simulink model "SWC_FDC_type"  (R2021b)
settings: Solver=FixedStepDiscrete  StartTime=0.0  StopTime=10.0  FixedStep=0.001  RelTol=1e-3
values from neighbouring files (symbols this model uses):
  C_TASK_5MS_S = (	C_TICK_TIME_S      	)    [vcu_local_hdr.m]
  DID_VCUKey = uint16(0x0202)    [vcu_local_hdr.m]
  DID_XWD = uint16(513)    [vcu_local_hdr.m]
  DIDLen_DKCKey = uint16(8)    [vcu_local_hdr.m]
  DIDLen_FoxPiBattSta = uint16(4)    [vcu_local_hdr.m]
  DIDLen_FoxPiBrakeSta = uint16(13)    [vcu_local_hdr.m]
  DIDLen_FoxPiButtonSta = uint16(2)    [vcu_local_hdr.m]
  DIDLen_FoxPiCtrlEnSw = uint16(1)    [vcu_local_hdr.m]
  DIDLen_FoxPiDrivingCtrl = uint16(21)    [vcu_local_hdr.m]
  DIDLen_FoxPiEPSSta = uint16(11)    [vcu_local_hdr.m]
  DIDLen_FoxPiLampCtrl = uint16(6)    [vcu_local_hdr.m]
  DIDLen_FoxPiLampSta = uint16(2)    [vcu_local_hdr.m]
  DIDLen_FoxPiMotionSta = uint16(13)    [vcu_local_hdr.m]
  DIDLen_FoxPiMotorSta = uint16(11)    [vcu_local_hdr.m]
  DIDLen_FoxPiPedalPos = uint16(3)    [vcu_local_hdr.m]
  DIDLen_FoxPiPTGUSSSw = uint16(1)    [vcu_local_hdr.m]
  DIDLen_FoxPiShifterAllow = uint16(3)    [vcu_local_hdr.m]
  DIDLen_FoxPiSwSta = uint16(2)    [vcu_local_hdr.m]
  DIDLen_FoxPiTPMSSta = uint16(13)    [vcu_local_hdr.m]
  DIDLen_FoxPiUSSDist = uint16(20)    [vcu_local_hdr.m]
  DIDLen_FoxPiUSSFaultSta = uint16(2)    [vcu_local_hdr.m]
  DIDLen_FoxPiWheelSpd = uint16(16)    [vcu_local_hdr.m]
  DIDNum_DKCKey = uint16(0x0202)    [vcu_local_hdr.m]
  DIDNum_FoxPiBattSta = uint16(0x100D)    [vcu_local_hdr.m]
  DIDNum_FoxPiBrakeSta = uint16(0x1003)    [vcu_local_hdr.m]
  DIDNum_FoxPiButtonSta = uint16(0x1006)    [vcu_local_hdr.m]
  DIDNum_FoxPiCtrlEnSw = uint16(0x1012)    [vcu_local_hdr.m]
  DIDNum_FoxPiDrivingCtrl = uint16(0x1001)    [vcu_local_hdr.m]
  DIDNum_FoxPiEPSSta = uint16(0x1005)    [vcu_local_hdr.m]
  DIDNum_FoxPiLampCtrl = uint16(0x100C)    [vcu_local_hdr.m]
  DIDNum_FoxPiLampSta = uint16(0x100B)    [vcu_local_hdr.m]
  DIDNum_FoxPiMotionSta = uint16(0x1002)    [vcu_local_hdr.m]
  DIDNum_FoxPiMotorSta = uint16(0x1010)    [vcu_local_hdr.m]
  DIDNum_FoxPiPedalPos = uint16(0x100F)    [vcu_local_hdr.m]
  DIDNum_FoxPiPTGUSSSw = uint16(0x1009)    [vcu_local_hdr.m]
  DIDNum_FoxPiShifterAllow = uint16(0x1011)    [vcu_local_hdr.m]
  DIDNum_FoxPiSwSta = uint16(0x100A)    [vcu_local_hdr.m]
  DIDNum_FoxPiTPMSSta = uint16(0x100E)    [vcu_local_hdr.m]
  DIDNum_FoxPiUSSDist = uint16(0x1007)    [vcu_local_hdr.m]
  DIDNum_FoxPiUSSFaultSta = uint16(0x1008)    [vcu_local_hdr.m]
  DIDNum_FoxPiWheelSpd = uint16(0x1004)    [vcu_local_hdr.m]
  DIDVCUKeyLength = uint16(8)    [vcu_local_hdr.m]
  DTC_10020B = Simulink.Parameter    [DTC_Constant_Definition.m]
  DTC_10020C = Simulink.Parameter    [DTC_Constant_Definition.m]
  DTC_10020D = Simulink.Parameter    [DTC_Constant_Definition.m]
  DTC_10020E = Simulink.Parameter    [DTC_Constant_Definition.m]
  DTC_100210 = Simulink.Parameter    [DTC_Constant_Definition.m]
  DTC_100211 = Simulink.Parameter    [DTC_Constant_Definition.m]
  DTC_100212 = Simulink.Parameter    [DTC_Constant_Definition.m]
  DTC_100213 = Simulink.Parameter    [DTC_Constant_Definition.m]
  DTC_100214 = Simulink.Parameter    [DTC_Constant_Definition.m]
  DTC_100215 = Simulink.Parameter    [DTC_Constant_Definition.m]
  DTC_100216 = Simulink.Parameter    [DTC_Constant_Definition.m]
  DTC_100217 = Simulink.Parameter    [DTC_Constant_Definition.m]
  DTC_100218 = Simulink.Parameter    [DTC_Constant_Definition.m]
  DTC_100219 = Simulink.Parameter    [DTC_Constant_Definition.m]
  DTC_10021A = Simulink.Parameter    [DTC_Constant_Definition.m]
  DTC_10021B = Simulink.Parameter    [DTC_Constant_Definition.m]
  DTC_10021C = Simulink.Parameter    [DTC_Constant_Definition.m]
  DTC_10021D = Simulink.Parameter    [DTC_Constant_Definition.m]
  DTC_10021E = Simulink.Parameter    [DTC_Constant_Definition.m]
  DTC_100220 = Simulink.Parameter    [DTC_Constant_Definition.m]
  DTC_100221 = Simulink.Parameter    [DTC_Constant_Definition.m]
  DTC_100223 = Simulink.Parameter    [DTC_Constant_Definition.m]
  DTC_100224 = Simulink.Parameter    [DTC_Constant_Definition.m]
  DTC_100225 = Simulink.Parameter    [DTC_Constant_Definition.m]
  DTC_100226 = Simulink.Parameter    [DTC_Constant_Definition.m]
  DTC_100227 = Simulink.Parameter    [DTC_Constant_Definition.m]
  DTC_100242 = Simulink.Parameter    [DTC_Constant_Definition.m]
  DTC_100243 = Simulink.Parameter    [DTC_Constant_Definition.m]
  DTC_100244 = Simulink.Parameter    [DTC_Constant_Definition.m]
  DTC_100247 = Simulink.Parameter    [DTC_Constant_Definition.m]
  DTC_100248 = Simulink.Parameter    [DTC_Constant_Definition.m]
  DTC_100249 = Simulink.Parameter    [DTC_Constant_Definition.m]
  DTC_100250 = Simulink.Parameter    [DTC_Constant_Definition.m]
  DTC_100251 = Simulink.Parameter    [DTC_Constant_Definition.m]
  DTC_100252 = Simulink.Parameter    [DTC_Constant_Definition.m]
  DTC_100A10 = Simulink.Parameter    [DTC_Constant_Definition.m]
  DTC_100A12 = Simulink.Parameter    [DTC_Constant_Definition.m]
  DTC_100A16 = Simulink.Parameter    [DTC_Constant_Definition.m]
  DTC_100A17 = Simulink.Parameter    [DTC_Constant_Definition.m]
  DTC_100A18 = Simulink.Parameter    [DTC_Constant_Definition.m]
  DTC_100A19 = Simulink.Parameter    [DTC_Constant_Definition.m]
  DTC_500B01 = Simulink.Parameter    [DTC_Constant_Definition.m]
  DTC_500B02 = Simulink.Parameter    [DTC_Constant_Definition.m]
  DTC_500B03 = Simulink.Parameter    [DTC_Constant_Definition.m]
  DTC_500B04 = Simulink.Parameter    [DTC_Constant_Definition.m]
  DTC_500B05 = Simulink.Parameter    [DTC_Constant_Definition.m]
  DTC_500B06 = Simulink.Parameter    [DTC_Constant_Definition.m]
  DTC_500B07 = Simulink.Parameter    [DTC_Constant_Definition.m]
  DTC_500B08 = Simulink.Parameter    [DTC_Constant_Definition.m]
  DTC_500B09 = Simulink.Parameter    [DTC_Constant_Definition.m]
  DTC_500B0A = Simulink.Parameter    [DTC_Constant_Definition.m]
  DTC_500B0B = Simulink.Parameter    [DTC_Constant_Definition.m]
  DTC_500B0C = Simulink.Parameter    [DTC_Constant_Definition.m]
  DTC_500B0D = Simulink.Parameter    [DTC_Constant_Definition.m]
  DTC_500B0E = Simulink.Parameter    [DTC_Constant_Definition.m]
  DTC_500B0F = Simulink.Parameter    [DTC_Constant_Definition.m]
  DTC_500B10 = Simulink.Parameter    [DTC_Constant_Definition.m]
  DTC_90021F = Simulink.Parameter    [DTC_Constant_Definition.m]
  DTC_90022F = Simulink.Parameter    [DTC_Constant_Definition.m]
  DTC_900253 = Simulink.Parameter    [DTC_Constant_Definition.m]
  DTC_900254 = Simulink.Parameter    [DTC_Constant_Definition.m]
  DTC_900301 = Simulink.Parameter    [DTC_Constant_Definition.m]
  DTC_900302 = Simulink.Parameter    [DTC_Constant_Definition.m]
  DTC_900303 = Simulink.Parameter    [DTC_Constant_Definition.m]
  DTC_900304 = Simulink.Parameter    [DTC_Constant_Definition.m]
  DTC_900305 = Simulink.Parameter    [DTC_Constant_Definition.m]
  DTC_900909 = Simulink.Parameter    [DTC_Constant_Definition.m]
  DTC_90090A = Simulink.Parameter    [DTC_Constant_Definition.m]
  DTC_90090B = Simulink.Parameter    [DTC_Constant_Definition.m]
  DTC_90090C = Simulink.Parameter    [DTC_Constant_Definition.m]
  DTC_90090D = Simulink.Parameter    [DTC_Constant_Definition.m]
  DTC_90090E = Simulink.Parameter    [DTC_Constant_Definition.m]
  DTC_90090F = Simulink.Parameter    [DTC_Constant_Definition.m]
  DTC_900910 = Simulink.Parameter    [DTC_Constant_Definition.m]
  DTC_900911 = Simulink.Parameter    [DTC_Constant_Definition.m]
  DTC_900912 = Simulink.Parameter    [DTC_Constant_Definition.m]
  DTC_900913 = Simulink.Parameter    [DTC_Constant_Definition.m]
  DTC_900914 = Simulink.Parameter    [DTC_Constant_Definition.m]
  ... (+54 more)
undefined symbols (not defined in the file or in its folder): f32_ApsOutVehSpdSig, KHAL_CANBusOffDebounce_cnt, KHAL_CANBusOffDebounce_s, KHAL_DKCDecryptEnable_flg_ovrdflg, KHAL_DKCDecryptEnable_flg_ovrdval, KHAL_RandomNumberY1_enum, KHAL_RandomNumberY2_enum, KHAL_RandomNumberY_ovrdflg, KHAL_TPMSRESBUTT_flg_ovrdflg, KHAL_TPMSRESBUTT_flg_ovrdval, KINP_ReadVinCode_flg, P_boolean, R_DIDWriteCDD_CSOP_DIDSet_DKCKey, R_DIDWriteCDD_CSOP_DIDSet_FoxPiBattSta, R_DIDWriteCDD_CSOP_DIDSet_FoxPiBrakeSta, R_DIDWriteCDD_CSOP_DIDSet_FoxPiButtonSta, R_DIDWriteCDD_CSOP_DIDSet_FoxPiCtrlEnSw, R_DIDWriteCDD_CSOP_DIDSet_FoxPiDrivingCtrl, R_DIDWriteCDD_CSOP_DIDSet_FoxPiEPSSta, R_DIDWriteCDD_CSOP_DIDSet_FoxPiLampCtrl, R_DIDWriteCDD_CSOP_DIDSet_FoxPiLampSta, R_DIDWriteCDD_CSOP_DIDSet_FoxPiMotionSta, R_DIDWriteCDD_CSOP_DIDSet_FoxPiMotorSta, R_DIDWriteCDD_CSOP_DIDSet_FoxPiPedalPos, R_DIDWriteCDD_CSOP_DIDSet_FoxPiPTGUSSSw, R_DIDWriteCDD_CSOP_DIDSet_FoxPiShifterAllow, R_DIDWriteCDD_CSOP_DIDSet_FoxPiSwSta, R_DIDWriteCDD_CSOP_DIDSet_FoxPiTPMSSta, R_DIDWriteCDD_CSOP_DIDSet_FoxPiUSSDist, R_DIDWriteCDD_CSOP_DIDSet_FoxPiUSSFaultSta, R_DIDWriteCDD_CSOP_DIDSet_FoxPiWheelSpd, R_E2E_CAN3_VCU1_CSOP_Write_CAN3_VCU1, R_E2E_CAN3_VCU1_toNIDEC_CSOP_Write_CAN3_VCU1_toNIDEC, R_E2E_CAN4_VCU1_CSOP_Write_CAN4_VCU1, R_FDCCDD_Inner_CSOP_FDC_AppCallSleep, R_HALIN_IMU_CSOP_IMUSetSta, R_HALINCDD_CSOP_PAS_Handler, R_HALINCDD_CSOP_ResetPedalZeroPosDone, R_HALINCDD_CSOP_TPMSSensorIDRegSetResults, R_HALINCDD_CSOP_UDS_Main, R_HALOUT_APS_CSOP_ApsOutput, R_HALOUTCDD_CSOP_AppNmStateReq, R_HALOUTCDD_CSOP_IVIReset, R_HALOUTCDD_CSOP_SetAcoreRebootCmdACK, R_HALOUTCDD_CSOP_SetSysPwrStat ... (+80)
libraries: FVT_lib x447, simulink x289, hcu_lib x19, hdlsllib x9, app x1, halin x1, halout x1, matrix_library x1, inp x1, outp x1
(part 4 of 15)

== system SWC_FDC_type/run_SWC_FDC_Tx_1000ms_sys ==
  IRV_ms1000_CAN3_SG_GW_IVI6_toNIDEC_read : Inport
  function : TriggerPort  TriggerType=function-call  VariantControl=(inherit)  SampleTimeType=periodic  SampleTime=-1
  P_CAN3_GW_IVI6_toNIDEC_CAN3_SG_GW_IVI6_toNIDEC_write : Outport
  wires:
  IRV_ms1000_CAN3_SG_GW_IVI6_toNIDEC_read/1 -> P_CAN3_GW_IVI6_toNIDEC_CAN3_SG_GW_IVI6_toNIDEC_write/1

== system SWC_FDC_type/run_SWC_FDC_Tx_100ms_sys ==
  IRV_ms100_CAN1_SG_FD1_THCM1_read : Inport
  IRV_ms100_CAN3_SG_FD3_THCM1_read : Inport  Port=2
  function : TriggerPort  TriggerType=function-call  VariantControl=(inherit)  SampleTimeType=periodic  SampleTime=-1
  P_CAN1_FD1_THCM1_CAN1_SG_FD1_THCM1_write : Outport
  P_CAN3_FD3_THCM1_CAN3_SG_FD3_THCM1_write : Outport  Port=2
  wires:
  IRV_ms100_CAN1_SG_FD1_THCM1_read/1 -> P_CAN1_FD1_THCM1_CAN1_SG_FD1_THCM1_write/1
  IRV_ms100_CAN3_SG_FD3_THCM1_read/1 -> P_CAN3_FD3_THCM1_CAN3_SG_FD3_THCM1_write/1

== system SWC_FDC_type/run_SWC_FDC_Tx_10ms_sys ==
  IRV_ms10_CAN1_SG_FD1_APS3_read : Inport
  IRV_ms10_CAN1_SG_FD1_VCU2_read : Inport  Port=2
  IRV_ms10_CAN1_SG_FD1_VCU3_read : Inport  Port=3
  IRV_ms10_CAN1_SG_VMC_FCM1_read : Inport  Port=4
  IRV_ms10_CAN3_SG_FD3_VCU0_read : Inport  Port=5
  IRV_ms10_CAN3_SG_FD3_VCU2_read : Inport  Port=6
  IRV_ms10_CAN3_SG_FD3_VCU2_toNIDEC_read : Inport  Port=7
  IRV_ms10_CAN3_SG_FD3_VCU5_read : Inport  Port=8
  IRV_ms10_CAN3_SG_GW_ESC1_toNIDEC_read : Inport  Port=9
  IRV_ms10_CAN5_SG_FD5_Debug3_read : Inport  Port=10
  IRV_ms10_CAN6_SG_FD6_APS3_read : Inport  Port=11
  IRV_ms10_CAN6_SG_FD6_VCU2_read : Inport  Port=12
  IRV_f32_ApsOutVehSpdSig_read : Inport  Port=13
  IRV_u8_ApsOutGearPosnSig_read : Inport  Port=14
  IRV_u8_ApsOutSendChrgPlugSta_read : Inport  Port=15
  IRV_u8_ApsOutSetFrSensorOnCmd_read : Inport  Port=16
  IRV_u8_ApsOutSetFrSensorSwTOCmd_read : Inport  Port=17
  IRV_u8_ApsOutSetVehSpdTOCmd_read : Inport  Port=18
  function : TriggerPort  TriggerType=function-call  VariantControl=(inherit)  SampleTimeType=periodic  SampleTime=-1
  R_HALINCDD_CSOP_TPMS_GetRawData : FunctionCaller  FunctionPrototype=[u8_TPMSDataInSta,u8Array9_TPMSData] = R_HALINCDD_CSOP_TPMS_GetRawData()  OutputArgumentSpecifications=P_boolean, uint8([1;1;1;1;1;1;1;1;1])
  R_HALIN_APS_CSOP_ApsGetDist : FunctionCaller  FunctionPrototype=[u8Array8_PasInDist,u16Array4_ApsInDist] = R_HALIN_APS_CSOP_ApsGetDist()  OutputArgumentSpecifications=uint8([1;1;1;1;1;1;1;1]), uint16([1;1;1;1])
  R_HALIN_APS_CSOP_ApsGetDistLevel : FunctionCaller  FunctionPrototype=u8Array8_ApsInLevel = R_HALIN_APS_CSOP_ApsGetDistLevel()  OutputArgumentSpecifications=uint8([1;1;1;1;1;1;1;1])
  R_HALIN_APS_CSOP_ApsGetOtherStatus : FunctionCaller  FunctionPrototype=[u8_ApsInPASChime,u8_ApsInSensorLayout,u8_ApsInSysFailSta,u8_ApsInSysMode] = R_HALIN_APS_CSOP_ApsGetOtherStatus()  OutputArgumentSpecifications=uint8(1), uint8(1), uint8(1), uint8(1)
  R_HALIN_APS_CSOP_ApsGetUssSta : FunctionCaller  FunctionPrototype=u8Array12_ApsInUssSta = R_HALIN_APS_CSOP_ApsGetUssSta()  OutputArgumentSpecifications=uint8([1;1;1;1;1;1;1;1;1;1;1;1])
  R_HALOUT_APS_CSOP_ApsOutput : FunctionCaller  FunctionPrototype=R_HALOUT_APS_CSOP_ApsOutput(f32_ApsOutVehSpdSig,u8_ApsOutGearPosnSig,u8_ApsOutSetFrSensorOnCmd,u8_ApsOutSetVehSpdTOCmd,u8_ApsOutSetFrSensorSwTOCmd,u8_ApsOutSendChrgPlugSta)  InputArgumentSpecifications=single(1), uint8(1), uint8(1), uint8(1), uint8(1), uint8(1)
  P_CAN1_FD1_APS3_CAN1_SG_FD1_APS3_write : Outport
  P_CAN1_FD1_VCU2_CAN1_SG_FD1_VCU2_write : Outport  Port=2
  P_CAN1_FD1_VCU3_CAN1_SG_FD1_VCU3_write : Outport  Port=3
  P_CAN1_VMC_FCM1_CAN1_SG_VMC_FCM1_write : Outport  Port=4
  P_CAN3_FD3_VCU0_CAN3_SG_FD3_VCU0_write : Outport  Port=5
  P_CAN3_FD3_VCU2_CAN3_SG_FD3_VCU2_write : Outport  Port=6
  P_CAN3_FD3_VCU2_toNIDEC_CAN3_SG_FD3_VCU2_toNIDEC_write : Outport  Port=7
  P_CAN3_FD3_VCU5_CAN3_SG_FD3_VCU5_write : Outport  Port=8
  P_CAN3_GW_ESC1_toNIDEC_CAN3_SG_GW_ESC1_toNIDEC_write : Outport  Port=9
  P_CAN5_FD5_Debug3_CAN5_SG_FD5_Debug3_write : Outport  Port=10
  P_CAN6_FD6_APS3_CAN6_SG_FD6_APS3_write : Outport  Port=11
  P_CAN6_FD6_VCU2_CAN6_SG_FD6_VCU2_write : Outport  Port=12
  IRV_u16Array4_ApsInDist_write : Outport  Port=13  OutDataTypeStr=uint16  PortDimensions=4
  IRV_u8Array12_ApsInUssSta_write : Outport  Port=14  OutDataTypeStr=uint8  PortDimensions=12
  IRV_u8Array8_ApsInLevel_write : Outport  Port=15  OutDataTypeStr=uint8  PortDimensions=8
  IRV_u8Array8_PasInDist_write : Outport  Port=16  OutDataTypeStr=uint8  PortDimensions=8
  IRV_u8Array9_TPMSData_write : Outport  Port=17  OutDataTypeStr=uint8  PortDimensions=9
  IRV_u8_ApsInPASChime_write : Outport  Port=18  OutDataTypeStr=uint8  PortDimensions=1
  IRV_u8_ApsInSensorLayout_write : Outport  Port=19  OutDataTypeStr=uint8  PortDimensions=1
  IRV_u8_ApsInSysFailSta_write : Outport  Port=20  OutDataTypeStr=uint8  PortDimensions=1
  IRV_u8_ApsInSysMode_write : Outport  Port=21  OutDataTypeStr=uint8  PortDimensions=1
  IRV_u8_TPMSDataInSta_write : Outport  Port=22  OutDataTypeStr=uint8  PortDimensions=1
  wires:
  R_HALIN_APS_CSOP_ApsGetDist/1 -> IRV_u8Array8_PasInDist_write/1
  R_HALIN_APS_CSOP_ApsGetDist/2 -> IRV_u16Array4_ApsInDist_write/1
  R_HALIN_APS_CSOP_ApsGetDistLevel/1 -> IRV_u8Array8_ApsInLevel_write/1
  R_HALIN_APS_CSOP_ApsGetUssSta/1 -> IRV_u8Array12_ApsInUssSta_write/1
  IRV_f32_ApsOutVehSpdSig_read/1 -> R_HALOUT_APS_CSOP_ApsOutput/1
  IRV_u8_ApsOutGearPosnSig_read/1 -> R_HALOUT_APS_CSOP_ApsOutput/2
  IRV_u8_ApsOutSetFrSensorOnCmd_read/1 -> R_HALOUT_APS_CSOP_ApsOutput/3
  IRV_u8_ApsOutSetVehSpdTOCmd_read/1 -> R_HALOUT_APS_CSOP_ApsOutput/4
  IRV_u8_ApsOutSetFrSensorSwTOCmd_read/1 -> R_HALOUT_APS_CSOP_ApsOutput/5
  IRV_u8_ApsOutSendChrgPlugSta_read/1 -> R_HALOUT_APS_CSOP_ApsOutput/6
  R_HALIN_APS_CSOP_ApsGetOtherStatus/1 -> IRV_u8_ApsInPASChime_write/1
  R_HALIN_APS_CSOP_ApsGetOtherStatus/2 -> IRV_u8_ApsInSensorLayout_write/1
  R_HALIN_APS_CSOP_ApsGetOtherStatus/3 -> IRV_u8_ApsInSysFailSta_write/1
  R_HALIN_APS_CSOP_ApsGetOtherStatus/4 -> IRV_u8_ApsInSysMode_write/1
  R_HALINCDD_CSOP_TPMS_GetRawData/1 -> IRV_u8_TPMSDataInSta_write/1
  R_HALINCDD_CSOP_TPMS_GetRawData/2 -> IRV_u8Array9_TPMSData_write/1
  IRV_ms10_CAN1_SG_FD1_APS3_read/1 -> P_CAN1_FD1_APS3_CAN1_SG_FD1_APS3_write/1
  IRV_ms10_CAN1_SG_FD1_VCU2_read/1 -> P_CAN1_FD1_VCU2_CAN1_SG_FD1_VCU2_write/1
  IRV_ms10_CAN1_SG_FD1_VCU3_read/1 -> P_CAN1_FD1_VCU3_CAN1_SG_FD1_VCU3_write/1
  IRV_ms10_CAN1_SG_VMC_FCM1_read/1 -> P_CAN1_VMC_FCM1_CAN1_SG_VMC_FCM1_write/1
  IRV_ms10_CAN3_SG_FD3_VCU0_read/1 -> P_CAN3_FD3_VCU0_CAN3_SG_FD3_VCU0_write/1
  IRV_ms10_CAN3_SG_FD3_VCU2_toNIDEC_read/1 -> P_CAN3_FD3_VCU2_toNIDEC_CAN3_SG_FD3_VCU2_toNIDEC_write/1
  IRV_ms10_CAN3_SG_FD3_VCU5_read/1 -> P_CAN3_FD3_VCU5_CAN3_SG_FD3_VCU5_write/1
  IRV_ms10_CAN3_SG_GW_ESC1_toNIDEC_read/1 -> P_CAN3_GW_ESC1_toNIDEC_CAN3_SG_GW_ESC1_toNIDEC_write/1
  IRV_ms10_CAN5_SG_FD5_Debug3_read/1 -> P_CAN5_FD5_Debug3_CAN5_SG_FD5_Debug3_write/1
  IRV_ms10_CAN6_SG_FD6_APS3_read/1 -> P_CAN6_FD6_APS3_CAN6_SG_FD6_APS3_write/1
  IRV_ms10_CAN6_SG_FD6_VCU2_read/1 -> P_CAN6_FD6_VCU2_CAN6_SG_FD6_VCU2_write/1
  IRV_ms10_CAN3_SG_FD3_VCU2_read/1 -> P_CAN3_FD3_VCU2_CAN3_SG_FD3_VCU2_write/1

== system SWC_FDC_type/run_SWC_FDC_Tx_20ms_sys ==
  IRV_ms20_CAN1_SG_FD1_APS2_read : Inport
  IRV_ms20_CAN2_SG_FD2_C20_0_read : Inport  Port=2
  function : TriggerPort  TriggerType=function-call  VariantControl=(inherit)  SampleTimeType=periodic  SampleTime=-1
  P_CAN1_FD1_APS2_CAN1_SG_FD1_APS2_write : Outport
  P_CAN2_FD2_C20_0_CAN2_SG_FD2_C20_0_write : Outport  Port=2
  wires:
  IRV_ms20_CAN1_SG_FD1_APS2_read/1 -> P_CAN1_FD1_APS2_CAN1_SG_FD1_APS2_write/1
  IRV_ms20_CAN2_SG_FD2_C20_0_read/1 -> P_CAN2_FD2_C20_0_CAN2_SG_FD2_C20_0_write/1

== system SWC_FDC_type/run_SWC_FDC_Tx_5000ms_sys ==
  IRV_ms5000_CAN2_SG_FD2_Version_read : Inport
  function : TriggerPort  TriggerType=function-call  VariantControl=(inherit)  SampleTimeType=periodic  SampleTime=-1
  P_CAN2_FD2_Version_CAN2_SG_FD2_Version_write : Outport
  wires:
  IRV_ms5000_CAN2_SG_FD2_Version_read/1 -> P_CAN2_FD2_Version_CAN2_SG_FD2_Version_write/1

== system SWC_FDC_type/run_SWC_FDC_Tx_500ms_sys ==
  IRV_ms500_CAN1_SG_FD1_VMC2_read : Inport
  function : TriggerPort  TriggerType=function-call  VariantControl=(inherit)  SampleTimeType=periodic  SampleTime=-1
  P_CAN1_FD1_VMC2_CAN1_SG_FD1_VMC2_write : Outport
  wires:
  IRV_ms500_CAN1_SG_FD1_VMC2_read/1 -> P_CAN1_FD1_VMC2_CAN1_SG_FD1_VMC2_write/1

== system SWC_FDC_type/run_SWC_FDC_UDS_10ms_sys ==
  function : TriggerPort  TriggerType=function-call  VariantControl=(inherit)  SampleTimeType=periodic  SampleTime=-1
  R_HALINCDD_CSOP_UDS_Main : FunctionCaller  FunctionPrototype=R_HALINCDD_CSOP_UDS_Main()

== system SWC_FDC_type/P_WDGCDD/run_SWC_FDC_AppCallWDG_End_sys ==
  function : TriggerPort  TriggerType=function-call  IsSimulinkFunction=on  FunctionName=run_SWC_FDC_AppCallWDG_End  VariantControl=(inherit)

== system SWC_FDC_type/P_WDGCDD/run_SWC_FDC_AppCallWDG_StartUp_sys ==
  function : TriggerPort  TriggerType=function-call  IsSimulinkFunction=on  FunctionName=run_SWC_FDC_AppCallWDG_StartUp  VariantControl=(inherit)

== system SWC_FDC_type/P_WDGCDD/run_SWC_FDC_AppCallWDG_sys ==
  function : TriggerPort  TriggerType=function-call  IsSimulinkFunction=on  FunctionName=run_SWC_FDC_AppCallWDG  VariantControl=(inherit)

== system SWC_FDC_type/run_SWC_FDC_RxTx_5ms_sys/DIDGet_Subsystem ==
  trig_GetDID : TriggerPort  TriggerType=function-call  VariantControl=(inherit)  PortDimensions=1
  DIDLen : Constant  Value=DIDNum_DKCKey
  DIDLen1 : Constant  Value=DIDNum_FoxPiDrivingCtrl
  DIDLen2 : Constant  Value=DIDNum_FoxPiLampCtrl
  DIDLen3 : Constant  Value=DIDNum_FoxPiCtrlEnSw
  DIDNum : Constant  Value=DIDLen_DKCKey
  DIDNum1 : Constant  Value=DIDLen_FoxPiDrivingCtrl
  DIDNum2 : Constant  Value=DIDLen_FoxPiLampCtrl
  DIDNum3 : Constant  Value=DIDLen_FoxPiCtrlEnSw
  R_DIDReadCDD_CSOP_DIDGet_DKCKey : FunctionCaller  FunctionPrototype=[u8Array8_DKCKey,u8_DIDSta_DKCKey] = R_DIDReadCDD_CSOP_DIDGet_DKCKey(u16_DIDNum_DKCKey,u16_DIDLen_DKCKey)  InputArgumentSpecifications=uint16(1), uint16(1)  OutputArgumentSpecifications=uint8([1;1;1;1;1;1;1;1]), uint8(1)
  R_DIDReadCDD_CSOP_DIDGet_FoxPiCtrlEnSw : FunctionCaller  FunctionPrototype=[u8_FoxPiCtrlEnSw,u8_DIDSta_FoxPiCtrlEnSw] = R_DIDReadCDD_CSOP_DIDGet_FoxPiCtrlEnSw(u16_DIDNum_FoxPiCtrlEnSw,u16_DIDLen_FoxPiCtrlEnSw)  InputArgumentSpecifications=uint16(1), uint16(1)  OutputArgumentSpecifications=uint8(1), uint8(1)
  R_DIDReadCDD_CSOP_DIDGet_FoxPiDrivingCtrl : FunctionCaller  FunctionPrototype=[u8Array21_FoxPiDrivingCtrl,u8_DIDSta_FoxPiDrivingCtrl] = R_DIDReadCDD_CSOP_DIDGet_FoxPiDrivingCtrl(u16_DIDNum_FoxPiDrivingCtrl,u16_DIDLen_FoxPiDrivingCtrl)  InputArgumentSpecifications=uint16(1), uint16(1)  OutputArgumentSpecifications=uint8([1;1;1;1;1;1;1;1;1;1;1;1;1;1;1;1;1;1;1;1;1]), uint8(1)
  R_DIDReadCDD_CSOP_DIDGet_FoxPiLampCtrl : FunctionCaller  FunctionPrototype=[u8Array6_FoxPiLampCtrl,u8_DIDSta_FoxPiLampCtrl] = R_DIDReadCDD_CSOP_DIDGet_FoxPiLampCtrl(u16_DIDNum_FoxPiLampCtrl,u16_DIDLen_FoxPiLampCtrl)  InputArgumentSpecifications=uint16(1), uint16(1)  OutputArgumentSpecifications=uint8([1;1;1;1;1;1]), uint8(1)
  UnitConverter{,1..7} (8 alike) : DataTypeConversion  OutDataTypeStr=uint8
  bus_Creator : BusCreator  Inputs=8
  BHAL_DID_outputs : Outport
  wires:
  [u8_DIDSta_DKCKey] -> UnitConverter/1  "u8_DIDSta_DKCKey"
  UnitConverter/1 -> bus_Creator/1  "VHAL_DIDStaDKCKey_raw"
  [u8Array8_DKCKey] -> UnitConverter1/1  "u8Array8_DKCKey"
  UnitConverter1/1 -> bus_Creator/2  "VHAL_DKCKey_raw"
  [u8_DIDSta_FoxPiDrivingCtrl] -> UnitConverter2/1  "u8_DIDSta_FoxPiDrivingCtrl"
  UnitConverter2/1 -> bus_Creator/3  "VHAL_DIDStaFoxPiDrivingCtrl_raw"
  [u8Array19_FoxPiDrivingCtrl] -> UnitConverter3/1  "u8Array19_FoxPiDrivingCtrl"
  UnitConverter3/1 -> bus_Creator/4  "VHAL_FoxPiDrivingCtrl_raw"
  [u8_DIDSta_FoxPiLampCtrl] -> UnitConverter4/1  "u8_DIDSta_FoxPiLampCtrl"
  UnitConverter4/1 -> bus_Creator/5  "VHAL_DIDStaFoxPiLampCtrl_raw"
  [u8Array6_FoxPiLampCtrl] -> UnitConverter5/1  "u8Array6_FoxPiLampCtrl"
  UnitConverter5/1 -> bus_Creator/6  "VHAL_FoxPiLampCtrl_raw"
  [u8_DIDSta_FoxPiCtrlEnSw] -> UnitConverter6/1  "u8_DIDSta_FoxPiCtrlEnSw"
  UnitConverter6/1 -> bus_Creator/7  "VHAL_DIDStaFoxPiCtrlEnSw_raw"
  [u8_FoxPiCtrlEnSw] -> UnitConverter7/1  "u8_FoxPiCtrlEnSw"
  UnitConverter7/1 -> bus_Creator/8  "VHAL_FoxPiCtrlEnSw_raw"
  bus_Creator/1 -> BHAL_DID_outputs/1
  DIDLen/1 -> R_DIDReadCDD_CSOP_DIDGet_DKCKey/1
  DIDNum/1 -> R_DIDReadCDD_CSOP_DIDGet_DKCKey/2
  R_DIDReadCDD_CSOP_DIDGet_DKCKey/1 -> [u8Array8_DKCKey]
  R_DIDReadCDD_CSOP_DIDGet_DKCKey/2 -> [u8_DIDSta_DKCKey]
  DIDLen1/1 -> R_DIDReadCDD_CSOP_DIDGet_FoxPiDrivingCtrl/1
  DIDNum1/1 -> R_DIDReadCDD_CSOP_DIDGet_FoxPiDrivingCtrl/2
  R_DIDReadCDD_CSOP_DIDGet_FoxPiDrivingCtrl/1 -> [u8Array19_FoxPiDrivingCtrl]
  R_DIDReadCDD_CSOP_DIDGet_FoxPiDrivingCtrl/2 -> [u8_DIDSta_FoxPiDrivingCtrl]
  DIDLen2/1 -> R_DIDReadCDD_CSOP_DIDGet_FoxPiLampCtrl/1
  DIDNum2/1 -> R_DIDReadCDD_CSOP_DIDGet_FoxPiLampCtrl/2
  R_DIDReadCDD_CSOP_DIDGet_FoxPiLampCtrl/1 -> [u8Array6_FoxPiLampCtrl]
  R_DIDReadCDD_CSOP_DIDGet_FoxPiLampCtrl/2 -> [u8_DIDSta_FoxPiLampCtrl]
  DIDLen3/1 -> R_DIDReadCDD_CSOP_DIDGet_FoxPiCtrlEnSw/1
  DIDNum3/1 -> R_DIDReadCDD_CSOP_DIDGet_FoxPiCtrlEnSw/2
  R_DIDReadCDD_CSOP_DIDGet_FoxPiCtrlEnSw/1 -> [u8_FoxPiCtrlEnSw]
  R_DIDReadCDD_CSOP_DIDGet_FoxPiCtrlEnSw/2 -> [u8_DIDSta_FoxPiCtrlEnSw]

== system SWC_FDC_type/run_SWC_FDC_RxTx_5ms_sys/DIDSet_Subsystem ==
  BOUTP_DIDSetData_outputs : Inport
  BHAL_DID_outputs : Inport  Port=2
  trig_SetDID : TriggerPort  TriggerType=function-call  VariantControl=(inherit)  PortDimensions=1
  DIDLen : Constant  Value=DIDNum_DKCKey
  DIDLen1 : Constant  Value=DIDNum_FoxPiDrivingCtrl
  DIDLen10 : Constant  Value=DIDNum_FoxPiSwSta
  DIDLen11 : Constant  Value=DIDNum_FoxPiLampSta
  DIDLen12 : Constant  Value=DIDNum_FoxPiLampCtrl
  DIDLen13 : Constant  Value=DIDNum_FoxPiBattSta
  DIDLen14 : Constant  Value=DIDNum_FoxPiTPMSSta
  DIDLen15 : Constant  Value=DIDNum_FoxPiPedalPos
  DIDLen16 : Constant  Value=DIDNum_FoxPiMotorSta
  DIDLen17 : Constant  Value=DIDNum_FoxPiShifterAllow
  DIDLen18 : Constant  Value=DIDNum_FoxPiCtrlEnSw
  DIDLen2 : Constant  Value=DIDNum_FoxPiMotionSta
  DIDLen3 : Constant  Value=DIDNum_FoxPiBrakeSta
  DIDLen4 : Constant  Value=DIDNum_FoxPiWheelSpd
  DIDLen5 : Constant  Value=DIDNum_FoxPiEPSSta
  DIDLen6 : Constant  Value=DIDNum_FoxPiButtonSta
  DIDLen7 : Constant  Value=DIDNum_FoxPiUSSDist
  DIDLen8 : Constant  Value=DIDNum_FoxPiUSSFaultSta
  DIDLen9 : Constant  Value=DIDNum_FoxPiPTGUSSSw
  DIDNum : Constant  Value=DIDLen_DKCKey
  DIDNum1 : Constant  Value=DIDLen_FoxPiDrivingCtrl
  DIDNum10 : Constant  Value=DIDLen_FoxPiSwSta
  DIDNum11 : Constant  Value=DIDLen_FoxPiLampSta
  DIDNum12 : Constant  Value=DIDLen_FoxPiLampCtrl
  DIDNum13 : Constant  Value=DIDLen_FoxPiBattSta
  DIDNum14 : Constant  Value=DIDLen_FoxPiTPMSSta
  DIDNum15 : Constant  Value=DIDLen_FoxPiPedalPos
  DIDNum16 : Constant  Value=DIDLen_FoxPiMotorSta
  DIDNum17 : Constant  Value=DIDLen_FoxPiShifterAllow
  DIDNum18 : Constant  Value=DIDLen_FoxPiCtrlEnSw
  DIDNum2 : Constant  Value=DIDLen_FoxPiMotionSta
  DIDNum3 : Constant  Value=DIDLen_FoxPiBrakeSta
  DIDNum4 : Constant  Value=DIDLen_FoxPiWheelSpd
  DIDNum5 : Constant  Value=DIDLen_FoxPiEPSSta
  DIDNum6 : Constant  Value=DIDLen_FoxPiButtonSta
  DIDNum7 : Constant  Value=DIDLen_FoxPiUSSDist
  DIDNum8 : Constant  Value=DIDLen_FoxPiUSSFaultSta
  DIDNum9 : Constant  Value=DIDLen_FoxPiPTGUSSSw
  R_DIDWriteCDD_CSOP_DIDSet_DKCKey : FunctionCaller  FunctionPrototype=R_DIDWriteCDD_CSOP_DIDSet_DKCKey(u16_DIDNum_DKCKey,u16_DIDLen_DKCKey,u8Array8_DKCKey)  InputArgumentSpecifications=uint16(1), uint16(1), uint8([1;1;1;1;1;1;1;1])
  R_DIDWriteCDD_CSOP_DIDSet_FoxPiBattSta : FunctionCaller  FunctionPrototype=R_DIDWriteCDD_CSOP_DIDSet_FoxPiBattSta(u16_DIDNum_FoxPiBattSta,u16_DIDLen_FoxPiBattSta,u8Array4_FoxPiBattSta)  InputArgumentSpecifications=uint16(1), uint16(1), uint8([1;1;1;1])
  R_DIDWriteCDD_CSOP_DIDSet_FoxPiBrakeSta : FunctionCaller  FunctionPrototype=R_DIDWriteCDD_CSOP_DIDSet_FoxPiBrakeSta(u16_DIDNum_FoxPiBrakeSta,u16_DIDLen_FoxPiBrakeSta,u8Array13_FoxPiBrakeSta)  InputArgumentSpecifications=uint16(1), uint16(1), uint8([1;1;1;1;1;1;1;1;1;1;1;1;1])
  R_DIDWriteCDD_CSOP_DIDSet_FoxPiButtonSta : FunctionCaller  FunctionPrototype=R_DIDWriteCDD_CSOP_DIDSet_FoxPiButtonSta(u16_DIDNum_FoxPiButtonSta,u16_DIDLen_FoxPiButtonSta,u8Array2_FoxPiButtonSta)  InputArgumentSpecifications=uint16(1), uint16(1), uint8([1;1])
  R_DIDWriteCDD_CSOP_DIDSet_FoxPiCtrlEnSw : FunctionCaller  FunctionPrototype=R_DIDWriteCDD_CSOP_DIDSet_FoxPiCtrlEnSw(u16_DIDNum_FoxPiCtrlEnSw,u16_DIDLen_FoxPiCtrlEnSw,u8_FoxPiCtrlEnSw)  InputArgumentSpecifications=uint16(1), uint16(1), uint8(1)
  R_DIDWriteCDD_CSOP_DIDSet_FoxPiDrivingCtrl : FunctionCaller  FunctionPrototype=R_DIDWriteCDD_CSOP_DIDSet_FoxPiDrivingCtrl(u16_DIDNum_FoxPiDrivingCtrl,u16_DIDLen_FoxPiDrivingCtrl,u8Array21_FoxPiDrivingCtrl)  InputArgumentSpecifications=uint16(1), uint16(1), uint8([1;1;1;1;1;1;1;1;1;1;1;1;1;1;1;1;1;1;1;1;1])
  R_DIDWriteCDD_CSOP_DIDSet_FoxPiEPSSta : FunctionCaller  FunctionPrototype=R_DIDWriteCDD_CSOP_DIDSet_FoxPiEPSSta(u16_DIDNum_FoxPiEPSSta,u16_DIDLen_FoxPiEPSSta,u8Array11_FoxPiEPSSta)  InputArgumentSpecifications=uint16(1), uint16(1), uint8([1;1;1;1;1;1;1;1;1;1;1])
  R_DIDWriteCDD_CSOP_DIDSet_FoxPiLampCtrl : FunctionCaller  FunctionPrototype=R_DIDWriteCDD_CSOP_DIDSet_FoxPiLampCtrl(u16_DIDNum_FoxPiLampCtrl,u16_DIDLen_FoxPiLampCtrl,u8Array6_FoxPiLampCtrl)  InputArgumentSpecifications=uint16(1), uint16(1), uint8([1;1;1;1;1;1])
  R_DIDWriteCDD_CSOP_DIDSet_FoxPiLampSta : FunctionCaller  FunctionPrototype=R_DIDWriteCDD_CSOP_DIDSet_FoxPiLampSta(u16_DIDNum_FoxPiLampSta,u16_DIDLen_FoxPiLampSta,u8Array2_FoxPiLampSta)  InputArgumentSpecifications=uint16(1), uint16(1), uint8([1;1])
  R_DIDWriteCDD_CSOP_DIDSet_FoxPiMotionSta : FunctionCaller  FunctionPrototype=R_DIDWriteCDD_CSOP_DIDSet_FoxPiMotionSta(u16_DIDNum_FoxPiMotionSta,u16_DIDLen_FoxPiMotionSta,u8Array13_FoxPiMotionSta)  InputArgumentSpecifications=uint16(1), uint16(1), uint8([1;1;1;1;1;1;1;1;1;1;1;1;1])
  R_DIDWriteCDD_CSOP_DIDSet_FoxPiMotorSta : FunctionCaller  FunctionPrototype=R_DIDWriteCDD_CSOP_DIDSet_FoxPiMotorSta(u16_DIDNum_FoxPiMotorSta,u16_DIDLen_FoxPiMotorSta,u8Array11_FoxPiMotorSta)  InputArgumentSpecifications=uint16(1), uint16(1), uint8([1;1;1;1;1;1;1;1;1;1;1])
  R_DIDWriteCDD_CSOP_DIDSet_FoxPiPTGUSSSw : FunctionCaller  FunctionPrototype=R_DIDWriteCDD_CSOP_DIDSet_FoxPiPTGUSSSw(u16_DIDNum_FoxPiPTGUSSSw,u16_DIDLen_FoxPiPTGUSSSw,u8_FoxPiPTGUSSSw)  InputArgumentSpecifications=uint16(1), uint16(1), uint8(1)
  R_DIDWriteCDD_CSOP_DIDSet_FoxPiPedalPos : FunctionCaller  FunctionPrototype=R_DIDWriteCDD_CSOP_DIDSet_FoxPiPedalPos(u16_DIDNum_FoxPiPedalPos,u16_DIDLen_FoxPiPedalPos,u8Array3_FoxPiPedalPos)  InputArgumentSpecifications=uint16(1), uint16(1), uint8([1;1;1])
  R_DIDWriteCDD_CSOP_DIDSet_FoxPiShifterAllow : FunctionCaller  FunctionPrototype=R_DIDWriteCDD_CSOP_DIDSet_FoxPiShifterAllow(u16_DIDNum_FoxPiShifterAllow,u16_DIDLen_FoxPiShifterAllow,u8Array3_FoxPiShifterAllow)  InputArgumentSpecifications=uint16(1), uint16(1), uint8([1;1;1])
  R_DIDWriteCDD_CSOP_DIDSet_FoxPiSwSta : FunctionCaller  FunctionPrototype=R_DIDWriteCDD_CSOP_DIDSet_FoxPiSwSta(u16_DIDNum_FoxPiSwSta,u16_DIDLen_FoxPiSwSta,u8Array2_FoxPiSwSta)  InputArgumentSpecifications=uint16(1), uint16(1), uint8([1;1])
  R_DIDWriteCDD_CSOP_DIDSet_FoxPiTPMSSta : FunctionCaller  FunctionPrototype=R_DIDWriteCDD_CSOP_DIDSet_FoxPiTPMSSta(u16_DIDNum_FoxPiTPMSSta,u16_DIDLen_FoxPiTPMSSta,u8Array13_FoxPiTPMSSta)  InputArgumentSpecifications=uint16(1), uint16(1), uint8([1;1;1;1;1;1;1;1;1;1;1;1;1])
  R_DIDWriteCDD_CSOP_DIDSet_FoxPiUSSDist : FunctionCaller  FunctionPrototype=R_DIDWriteCDD_CSOP_DIDSet_FoxPiUSSDist(u16_DIDNum_FoxPiUSSDist,u16_DIDLen_FoxPiUSSDist,u8Array20_FoxPiUSSDist)  InputArgumentSpecifications=uint16(1), uint16(1), uint8([1;1;1;1;1;1;1;1;1;1;1;1;1;1;1;1;1;1;1;1])
  R_DIDWriteCDD_CSOP_DIDSet_FoxPiUSSFaultSta : FunctionCaller  FunctionPrototype=R_DIDWriteCDD_CSOP_DIDSet_FoxPiUSSFaultSta(u16_DIDNum_FoxPiUSSFaultSta,u16_DIDLen_FoxPiUSSFaultSta,u8Array2_FoxPiUSSFaultSta)  InputArgumentSpecifications=uint16(1), uint16(1), uint8([1;1])
  R_DIDWriteCDD_CSOP_DIDSet_FoxPiWheelSpd : FunctionCaller  FunctionPrototype=R_DIDWriteCDD_CSOP_DIDSet_FoxPiWheelSpd(u16_DIDNum_FoxPiWheelSpd,u16_DIDLen_FoxPiWheelSpd,u8Array16_FoxPiWheelSpd)  InputArgumentSpecifications=uint16(1), uint16(1), uint8([1;1;1;1;1;1;1;1;1;1;1;1;1;1;1;1])
  bus_selector : BusSelector  OutputSignals=VHAL_DIDSetFoxPiMotionSta_raw8,VHAL_DIDSetFoxPiBrakeSta_raw8,VHAL_DIDSetFoxPiWheelSpd_raw8,VHAL_DIDSetFoxPiEPSSta_raw8,VHAL_DIDSetFoxPiButtonSta_raw8,VHAL_DIDSetFoxPiUSSDist_raw8,VHAL_DIDSetFoxPiUSSFaultSta_raw8,VHAL_DIDSetFoxPiPTGUSSSw_raw8,VHAL_DIDSetFoxPiSwSta_raw8,VHAL_DIDSetFoxPiLampSta_raw8,VHAL_DIDSetFoxPiBattSta_raw8,VHAL_DIDSetFoxPiTPMSSta_raw8,VHAL_DIDSetFoxPiPedalPos_raw8,VHAL_DIDSetFoxPiMotorSta_raw8,VHAL_DIDSetFoxPiShifterAllow_raw8
  bus_selector1 : BusSelector  OutputSignals=VHAL_DIDStaDKCKey_raw,VHAL_DKCKey_raw,VHAL_DIDStaFoxPiDrivingCtrl_raw,VHAL_FoxPiDrivingCtrl_raw,VHAL_DIDStaFoxPiLampCtrl_raw,VHAL_FoxPiLampCtrl_raw,VHAL_DIDStaFoxPiCtrlEnSw_raw,VHAL_FoxPiCtrlEnSw_raw
  wires:
  bus_selector/1 -> [u8Array13_FoxPiMotionSta]  "<VHAL_DIDSetFoxPiMotionSta_raw8>"
  bus_selector/2 -> [u8Array13_FoxPiBrakeSta]  "<VHAL_DIDSetFoxPiBrakeSta_raw8>"
  bus_selector/3 -> [u8Array16_FoxPiWheelSpd]  "<VHAL_DIDSetFoxPiWheelSpd_raw8>"
  bus_selector/4 -> [u8Array11_FoxPiEPSSta]  "<VHAL_DIDSetFoxPiEPSSta_raw8>"
  bus_selector/5 -> [u8Array2_FoxPiButtonSta]  "<VHAL_DIDSetFoxPiButtonSta_raw8>"
  bus_selector/6 -> [u8Array20_FoxPiUSSDist]  "<VHAL_DIDSetFoxPiUSSDist_raw8>"
  bus_selector/7 -> [u8Array2_FoxPiUSSFaultSta]  "<VHAL_DIDSetFoxPiUSSFaultSta_raw8>"
  bus_selector/8 -> [u8_FoxPiPTGUSSSw]  "<VHAL_DIDSetFoxPiPTGUSSSw_raw8>"
  bus_selector/9 -> [u8Array2_FoxPiSwSta]  "<VHAL_DIDSetFoxPiSwSta_raw8>"
  bus_selector/10 -> [u8Array2_FoxPiLampSta]  "<VHAL_DIDSetFoxPiLampSta_raw8>"
  bus_selector/11 -> [u8Array4_FoxPiBattSta]  "<VHAL_DIDSetFoxPiBattSta_raw8>"
  bus_selector/12 -> [u8Array13_FoxPiTPMSSta]  "<VHAL_DIDSetFoxPiTPMSSta_raw8>"
  bus_selector/13 -> [u8Array3_FoxPiPedalPos]  "<VHAL_DIDSetFoxPiPedalPos_raw8>"
  bus_selector/14 -> [u8Array11_FoxPiMotorSta]  "<VHAL_DIDSetFoxPiMotorSta_raw8>"
  bus_selector/15 -> [u8Array3_FoxPiShifterAllow]  "<VHAL_DIDSetFoxPiShifterAllow_raw8>"
  BOUTP_DIDSetData_outputs/1 -> bus_selector/1
  bus_selector1/1 -> [u8_DIDSta_DKCKey]  "<VHAL_DIDStaDKCKey_raw>"
  bus_selector1/2 -> [u8Array8_DKCKey]  "<VHAL_DKCKey_raw>"
  bus_selector1/3 -> [u8_DIDSta_FoxPiDrivingCtrl]  "<VHAL_DIDStaFoxPiDrivingCtrl_raw>"
  bus_selector1/4 -> [u8Array19_FoxPiDrivingCtrl]  "<VHAL_FoxPiDrivingCtrl_raw>"
  bus_selector1/5 -> [u8_DIDSta_FoxPiLampCtrl]  "<VHAL_DIDStaFoxPiLampCtrl_raw>"
  bus_selector1/6 -> [u8Array6_FoxPiLampCtrl]  "<VHAL_FoxPiLampCtrl_raw>"
  bus_selector1/7 -> [u8_DIDSta_FoxPiCtrlEnSw]  "<VHAL_DIDStaFoxPiCtrlEnSw_raw>"
  bus_selector1/8 -> [u8_FoxPiCtrlEnSw]  "<VHAL_FoxPiCtrlEnSw_raw>"
  BHAL_DID_outputs/1 -> bus_selector1/1
  DIDLen/1 -> R_DIDWriteCDD_CSOP_DIDSet_DKCKey/1
  DIDNum/1 -> R_DIDWriteCDD_CSOP_DIDSet_DKCKey/2
  [u8Array8_DKCKey] -> R_DIDWriteCDD_CSOP_DIDSet_DKCKey/3
  DIDLen1/1 -> R_DIDWriteCDD_CSOP_DIDSet_FoxPiDrivingCtrl/1
  DIDNum1/1 -> R_DIDWriteCDD_CSOP_DIDSet_FoxPiDrivingCtrl/2
  [u8Array19_FoxPiDrivingCtrl] -> R_DIDWriteCDD_CSOP_DIDSet_FoxPiDrivingCtrl/3
  DIDLen2/1 -> R_DIDWriteCDD_CSOP_DIDSet_FoxPiMotionSta/1
  DIDNum2/1 -> R_DIDWriteCDD_CSOP_DIDSet_FoxPiMotionSta/2
  [u8Array13_FoxPiMotionSta] -> R_DIDWriteCDD_CSOP_DIDSet_FoxPiMotionSta/3
  DIDLen3/1 -> R_DIDWriteCDD_CSOP_DIDSet_FoxPiBrakeSta/1
  DIDNum3/1 -> R_DIDWriteCDD_CSOP_DIDSet_FoxPiBrakeSta/2
  [u8Array13_FoxPiBrakeSta] -> R_DIDWriteCDD_CSOP_DIDSet_FoxPiBrakeSta/3
  DIDLen4/1 -> R_DIDWriteCDD_CSOP_DIDSet_FoxPiWheelSpd/1
  DIDNum4/1 -> R_DIDWriteCDD_CSOP_DIDSet_FoxPiWheelSpd/2
  [u8Array16_FoxPiWheelSpd] -> R_DIDWriteCDD_CSOP_DIDSet_FoxPiWheelSpd/3
  DIDLen5/1 -> R_DIDWriteCDD_CSOP_DIDSet_FoxPiEPSSta/1
  DIDNum5/1 -> R_DIDWriteCDD_CSOP_DIDSet_FoxPiEPSSta/2
  [u8Array11_FoxPiEPSSta] -> R_DIDWriteCDD_CSOP_DIDSet_FoxPiEPSSta/3
  DIDLen6/1 -> R_DIDWriteCDD_CSOP_DIDSet_FoxPiButtonSta/1
  DIDNum6/1 -> R_DIDWriteCDD_CSOP_DIDSet_FoxPiButtonSta/2
  [u8Array2_FoxPiButtonSta] -> R_DIDWriteCDD_CSOP_DIDSet_FoxPiButtonSta/3
  DIDLen7/1 -> R_DIDWriteCDD_CSOP_DIDSet_FoxPiUSSDist/1
  DIDNum7/1 -> R_DIDWriteCDD_CSOP_DIDSet_FoxPiUSSDist/2
  [u8Array20_FoxPiUSSDist] -> R_DIDWriteCDD_CSOP_DIDSet_FoxPiUSSDist/3
  DIDLen8/1 -> R_DIDWriteCDD_CSOP_DIDSet_FoxPiUSSFaultSta/1
  DIDNum8/1 -> R_DIDWriteCDD_CSOP_DIDSet_FoxPiUSSFaultSta/2
  [u8Array2_FoxPiUSSFaultSta] -> R_DIDWriteCDD_CSOP_DIDSet_FoxPiUSSFaultSta/3
  DIDLen9/1 -> R_DIDWriteCDD_CSOP_DIDSet_FoxPiPTGUSSSw/1
  DIDNum9/1 -> R_DIDWriteCDD_CSOP_DIDSet_FoxPiPTGUSSSw/2
  [u8_FoxPiPTGUSSSw] -> R_DIDWriteCDD_CSOP_DIDSet_FoxPiPTGUSSSw/3
  DIDLen10/1 -> R_DIDWriteCDD_CSOP_DIDSet_FoxPiSwSta/1
  DIDNum10/1 -> R_DIDWriteCDD_CSOP_DIDSet_FoxPiSwSta/2
  [u8Array2_FoxPiSwSta] -> R_DIDWriteCDD_CSOP_DIDSet_FoxPiSwSta/3
  DIDLen11/1 -> R_DIDWriteCDD_CSOP_DIDSet_FoxPiLampSta/1
  DIDNum11/1 -> R_DIDWriteCDD_CSOP_DIDSet_FoxPiLampSta/2
  [u8Array2_FoxPiLampSta] -> R_DIDWriteCDD_CSOP_DIDSet_FoxPiLampSta/3
  DIDLen12/1 -> R_DIDWriteCDD_CSOP_DIDSet_FoxPiLampCtrl/1
  DIDNum12/1 -> R_DIDWriteCDD_CSOP_DIDSet_FoxPiLampCtrl/2
  [u8Array6_FoxPiLampCtrl] -> R_DIDWriteCDD_CSOP_DIDSet_FoxPiLampCtrl/3
  DIDLen13/1 -> R_DIDWriteCDD_CSOP_DIDSet_FoxPiBattSta/1
  DIDNum13/1 -> R_DIDWriteCDD_CSOP_DIDSet_FoxPiBattSta/2
  [u8Array4_FoxPiBattSta] -> R_DIDWriteCDD_CSOP_DIDSet_FoxPiBattSta/3
  DIDLen14/1 -> R_DIDWriteCDD_CSOP_DIDSet_FoxPiTPMSSta/1
  DIDNum14/1 -> R_DIDWriteCDD_CSOP_DIDSet_FoxPiTPMSSta/2
  [u8Array13_FoxPiTPMSSta] -> R_DIDWriteCDD_CSOP_DIDSet_FoxPiTPMSSta/3
  DIDLen15/1 -> R_DIDWriteCDD_CSOP_DIDSet_FoxPiPedalPos/1
  DIDNum15/1 -> R_DIDWriteCDD_CSOP_DIDSet_FoxPiPedalPos/2
  [u8Array3_FoxPiPedalPos] -> R_DIDWriteCDD_CSOP_DIDSet_FoxPiPedalPos/3
  DIDLen16/1 -> R_DIDWriteCDD_CSOP_DIDSet_FoxPiMotorSta/1
  DIDNum16/1 -> R_DIDWriteCDD_CSOP_DIDSet_FoxPiMotorSta/2
  [u8Array11_FoxPiMotorSta] -> R_DIDWriteCDD_CSOP_DIDSet_FoxPiMotorSta/3
  DIDLen17/1 -> R_DIDWriteCDD_CSOP_DIDSet_FoxPiShifterAllow/1
  DIDNum17/1 -> R_DIDWriteCDD_CSOP_DIDSet_FoxPiShifterAllow/2
  [u8Array3_FoxPiShifterAllow] -> R_DIDWriteCDD_CSOP_DIDSet_FoxPiShifterAllow/3
  DIDLen18/1 -> R_DIDWriteCDD_CSOP_DIDSet_FoxPiCtrlEnSw/1
  DIDNum18/1 -> R_DIDWriteCDD_CSOP_DIDSet_FoxPiCtrlEnSw/2
  [u8_FoxPiCtrlEnSw] -> R_DIDWriteCDD_CSOP_DIDSet_FoxPiCtrlEnSw/3

== system SWC_FDC_type/run_SWC_FDC_RxTx_5ms_sys/Function-Call Subsystem ==
  u8Array256_NvmReadArray : Inport
  function : TriggerPort  TriggerType=function-call  VariantControl=(inherit)
  u8Array256_NvmReadArrayInit : Outport
  wires:
  u8Array256_NvmReadArray/1 -> u8Array256_NvmReadArrayInit/1

== system SWC_FDC_type/run_SWC_FDC_RxTx_5ms_sys/HALOUT_AFTER ==
  E2E_CAN3_VCU1_Trigger : Inport
  E2E_CAN3_VCU1_Trigger_toNIDEC : Inport  Port=2
  E2E_CAN4_VCU1_Trigger : Inport  Port=3
  function : TriggerPort  TriggerType=function-call  VariantControl=(inherit)  PortDimensions=1
  R_E2E_CAN3_VCU1_CSOP_Write_CAN3_VCU1 : Subsystem
  R_E2E_CAN3_VCU1_toNIDEC_CSOP_Write_CAN3_VCU1_toNIDEC : Subsystem
  R_E2E_CAN4_VCU1_CSOP_Write_CAN4_VCU1 : Subsystem
  wires:
  E2E_CAN3_VCU1_Trigger/1 -> R_E2E_CAN3_VCU1_CSOP_Write_CAN3_VCU1/Enable
  E2E_CAN3_VCU1_Trigger_toNIDEC/1 -> R_E2E_CAN3_VCU1_toNIDEC_CSOP_Write_CAN3_VCU1_toNIDEC/Enable
  E2E_CAN4_VCU1_Trigger/1 -> R_E2E_CAN4_VCU1_CSOP_Write_CAN4_VCU1/Enable

== system SWC_FDC_type/run_SWC_FDC_RxTx_5ms_sys/Halin_CDD ==
  PASDistanceData : Inport
  APSDistanceData : Inport  Port=2
  APSLevelData : Inport  Port=3
  APSFaultStaData : Inport  Port=4
  ChimeIn : Inport  Port=5
  SNSRLayoutIn : Inport  Port=6
  StaFSyaIn : Inport  Port=7
  ModOperationIn : Inport  Port=8
  VHAL_AccelPedal1Vol_Raw : Inport  Port=9
  VHAL_AccelPedal2Vol_Raw : Inport  Port=10
  VHAL_BrakeSWGPIO_flg : Inport  Port=11
  VHAL_HoodSW_flg : Inport  Port=12
  VHAL_TailgateSW_flg : Inport  Port=13
  VHAL_DrDoorSW_flg : Inport  Port=14
  VHAL_PsDoorSW_flg : Inport  Port=15
  VHAL_RRDoorSW_flg : Inport  Port=16
  VHAL_RLDoorSW_flg : Inport  Port=17
  VHAL_CentralDoorLockSW_flg : Inport  Port=18
  VHAL_HazardSW_flg : Inport  Port=19
  VHAL_BrakeLampSW_flg : Inport  Port=20
  VHAL_TrunkHanSW_flg : Inport  Port=21
  VHAL_SeatSW_flg : Inport  Port=22
  VHAL_CrashSignalGPIO_flg : Inport  Port=23
  u8_HWID_4byte : Inport  Port=24
  u8_GetHWIDSta : Inport  Port=25
  GetSWID_status : Inport  Port=26
  GetSWID_data : Inport  Port=27
  VHAL_AnyNMID_flg : Inport  Port=28
  VHAL_CurrentNmState_enum : Inport  Port=29
  VHAL_PwrReq_OTA_enum : Inport  Port=30
  VHAL_AllowMovThd_OTA_enum : Inport  Port=31
  VHAL_EvccAplusPwrUpReq_flg : Inport  Port=32
  VHAL_AcoreReadyToSlp_flg : Inport  Port=33
  VHAL_DidXWDSta_flg : Inport  Port=34
  VHAL_DidXWDData_enum : Inport  Port=35
  HAL_NvmReadData_raw : Inport  Port=36
  VHAL_DIDVCUKeyReadSta_flg : Inport  Port=37
  VHAL_GetDIDVCUKey_enum : Inport  Port=38
  TPMS_DataIn_flg : Inport  Port=39
  TPMS_RawData : Inport  Port=40
  BHAL_CAN2_outputs : Inport  Port=41
  BHAL_CAN4_outputs : Inport  Port=42
  VHAL_ClearDTCcmd_flg : Inport  Port=43
  VHAL_IMUOffsetVal_raw : Inport  Port=44
  VHAL_IMUSixAxisVal_raw : Inport  Port=45
  VHAL_IMUOffsetValSta_flg : Inport  Port=46
  VHAL_IMUSixAxisValSta_flg : Inport  Port=47
  VHAL_NvmProtectSta_flg : Inport  Port=48
  VHAL_AuxBattVolmV_100mV : Inport  Port=49
  VHAL_Pedal1Ref5V_raw : Inport  Port=50
  VHAL_Pedal2Ref5V_raw : Inport  Port=51
  VHAL_NetworkReqCalled_flg : Inport  Port=52
  VHAL_PmicBootReason_enum : Inport  Port=53
  VHAL_WisrBootReason_raw32 : Inport  Port=54
  BHAL_DIDGetData_raw : Inport  Port=55
  VHAL_AcoreRebootCmd_raw : Inport  Port=56
  VHAL_CAN1BusOff_raw : Inport  Port=57
  VHAL_CAN2BusOff_raw : Inport  Port=58
  VHAL_CAN3BusOff_raw : Inport  Port=59
  VHAL_CAN4BusOff_raw : Inport  Port=60
  VHAL_CAN5BusOff_raw : Inport  Port=61
  VHAL_CAN6BusOff_raw : Inport  Port=62
  u8_GetAPS_Progress_PCT : Inport  Port=63
  u8_GetAPS_RQ_Display : Inport  Port=64
  u8_GetAPS_SW_Ver : Inport  Port=65
  u8_GetAPS_HW_Ver : Inport  Port=66
  u8_GetAPS_ExitCondition : Inport  Port=67
  f32_GetAPS_Angle_Target : Inport  Port=68
  u8_GetAPS_Sta_System : Inport  Port=69
  u8_GetAPS_V_Rq_EPAS_Ctrl : Inport  Port=70
  u8_GetAPS_Rq_EPAS_Ctrl : Inport  Port=71
  u8_GetAPS_Req : Inport  Port=72
  f32_GetAPS_DecReq : Inport  Port=73
  u8_GetAPS_DecReq_A : Inport  Port=74
  f32_GetAPS_SpeedCmd : Inport  Port=75
  u8_GetAPS_ShftPosnReq : Inport  Port=76
  u8_GetAPS_VMC_Req_A : Inport  Port=77
  u8_GetCAAS_Sta : Inport  Port=78
  u8_GetCAAS_VMC_Req_A : Inport  Port=79
  u8_TPMSSensorIDRegSta : Inport  Port=80
  u8_ResetPedalZeroPosReq : Inport  Port=81
  u8_GetAPS_PwrReq_cmd : Inport  Port=82
  u8_GetRAPS_BCM_LockReq_Cmd : Inport  Port=83
  u8_GetRAPS_BCM_Lamp_Cmd : Inport  Port=84
  u8_GetRAPS_ErrWarn_Sta : Inport  Port=85
  u8_GetRAPS_ErrLv1_flg : Inport  Port=86
  u32_BootPath : Inport  Port=87
  VHAL_CAN1RxErrorCount_raw : Inport  Port=88
  VHAL_CAN1TxErrorCount_raw : Inport  Port=89
  VHAL_CAN2RxErrorCount_raw : Inport  Port=90
  VHAL_CAN2TxErrorCount_raw : Inport  Port=91
  VHAL_CAN3RxErrorCount_cnt : Inport  Port=92
  VHAL_CAN3TxErrorCount_raw : Inport  Port=93
  VHAL_CAN4RxErrorCount_raw : Inport  Port=94
  VHAL_CAN4TxErrorCount_raw : Inport  Port=95
  VHAL_CAN5RxErrorCount_raw : Inport  Port=96
  VHAL_CAN5TxErrorCount_raw : Inport  Port=97
  VHAL_CAN6RxErrorCount_raw : Inport  Port=98
  VHAL_CAN6TxErrorCount_raw : Inport  Port=99
  trig_HalinCDD : TriggerPort  TriggerType=function-call  VariantControl=(inherit)
  Halin_APM : Subsystem
  Halin_DKC_A : Subsystem
  Halin_GPIO : Subsystem
  Halin_IMU : Subsystem
  Halin_SYS : Subsystem
  Halin_TPMS : Subsystem
  Subsystem : Subsystem
  TPM_Scheduler : Stateflow chart  TreatAsAtomicUnit=on
  BHAL_APM_outputs : Outport
  BHAL_GPIO_outputs : Outport  Port=2
  BHAL_SYS_outputs : Outport  Port=3
  BHAL_TPMS_outputs : Outport  Port=4
  BHAL_SYSTPMS_outputs : Outport  Port=5
  BHAL_DDM_outputs : Outport  Port=6
  BHAL_IMU_outputs : Outport  Port=7
  Enable_decrypt : Outport  Port=8
  AESKey : Outport  Port=9
  DKCRawData : Outport  Port=10
  wires:
  Halin_DKC_A/1(Enable_Decrypt) -> Enable_decrypt/1
  VHAL_RLDoorSW_flg/1 -> Halin_GPIO/9(VHAL_RLDoorSW_flg)
  Halin_SYS/1(BHAL_SYS_outputs) -> [BHAL_SYS_outputs], BHAL_SYS_outputs/1
  Halin_DKC_A/3(DKCRawData) -> DKCRawData/1
  GetSWID_data/1 -> Halin_SYS/2(GetSWID_data)
  VHAL_GetDIDVCUKey_enum/1 -> Halin_SYS/13(VHAL_GetDIDVCUKey_enum)
  VHAL_TailgateSW_flg/1 -> Halin_GPIO/5(VHAL_TailgateSW_flg)
  Halin_DKC_A/2(AESKey) -> AESKey/1
  VHAL_AccelPedal2Vol_Raw/1 -> Halin_GPIO/2(VHAL_AccelPedal2Vol_Raw)
  TPM_Scheduler/1(trig_TPM_10ms1()) -> Halin_TPMS/Trigger
  VHAL_TrunkHanSW_flg/1 -> Halin_GPIO/13(VHAL_TrunkHanSW_flg)
  VHAL_DidXWDSta_flg/1 -> Halin_SYS/9(VHAL_DidXWDSta_flg)
  VHAL_CurrentNmState_enum/1 -> Halin_SYS/4(VHAL_CurrentNmState_enum)
  VHAL_AccelPedal1Vol_Raw/1 -> Halin_GPIO/1(VHAL_AccelPedal1Vol_Raw)
  u8_HWID_4byte/1 -> Halin_GPIO/16(u8_HWID_4byte)
  BHAL_CAN2_outputs/1 -> Halin_TPMS/3(BHAL_CAN2_outputs)
  VHAL_AcoreReadyToSlp_flg/1 -> Halin_SYS/8(VHAL_AcoreReadyToSlp_flg)
  HAL_NvmReadData_raw/1 -> Halin_SYS/11(HAL_NvmReadData_raw)
  VHAL_AllowMovThd_OTA_enum/1 -> Halin_SYS/6(VHAL_AllowMovThd_OTA_enum)
  VHAL_BrakeLampSW_flg/1 -> Halin_GPIO/12(VHAL_BrakeLampSW_flg)
  VHAL_RRDoorSW_flg/1 -> Halin_GPIO/8(VHAL_RRDoorSW_flg)
  VHAL_BrakeSWGPIO_flg/1 -> Halin_GPIO/3(VHAL_BrakeSWGPIO_flg)
  GetSWID_status/1 -> Halin_SYS/1(GetSWID_status)
  VHAL_DrDoorSW_flg/1 -> Halin_GPIO/6(VHAL_DrDoorSW_flg)
  VHAL_PwrReq_OTA_enum/1 -> Halin_SYS/5(VHAL_PwrReq_OTA_enum)
  VHAL_HoodSW_flg/1 -> Halin_GPIO/4(VHAL_HoodSW_flg)
  Halin_GPIO/1(BHAL_GPIO_outputs) -> BHAL_GPIO_outputs/1
  BHAL_CAN4_outputs/1 -> Halin_DKC_A/1(BHAL_CAN4_outputs)
  VHAL_CentralDoorLockSW_flg/1 -> Halin_GPIO/10(VHAL_CentralDoorLockSW_flg)
  TPMS_RawData/1 -> Halin_TPMS/2(TPMS_RawData)
  VHAL_CrashSignalGPIO_flg/1 -> Halin_GPIO/15(VHAL_CrashSignalGPIO_flg)
  Halin_TPMS/1(BHAL_TPMS_outputs) -> BHAL_TPMS_outputs/1
  VHAL_DidXWDData_enum/1 -> Halin_SYS/10(VHAL_DidXWDData_enum)
  VHAL_EvccAplusPwrUpReq_flg/1 -> Halin_SYS/7(VHAL_EvccAplusPwrUpReq_flg)
  VHAL_SeatSW_flg/1 -> Halin_GPIO/14(VHAL_SeatSW_flg)
  VHAL_DIDVCUKeyReadSta_flg/1 -> Halin_SYS/12(VHAL_DIDVCUKeyReadSta_flg)
  VHAL_PsDoorSW_flg/1 -> Halin_GPIO/7(VHAL_PsDoorSW_flg)
  [BHAL_SYS_outputs] -> Halin_DKC_A/2(BHAL_SYS_outputs)
  TPMS_DataIn_flg/1 -> Halin_TPMS/1(TPMS_DataIn_flg)
  VHAL_AnyNMID_flg/1 -> Halin_SYS/3(VHAL_AnyNMID_flg)
  VHAL_HazardSW_flg/1 -> Halin_GPIO/11(VHAL_HazardSW_flg)
  Halin_SYS/2(BHAL_SYSTPMS_outputs) -> [BHAL_SYSTPMS_outputs], BHAL_SYSTPMS_outputs/1
  [BHAL_SYSTPMS_outputs] -> Halin_TPMS/4(BHAL_SYSTPMS_outputs)
  VHAL_ClearDTCcmd_flg/1 -> Subsystem/1(VHAL_ClearDTCcmd_flg)
  Subsystem/1(BHAL_DDM_outputs) -> BHAL_DDM_outputs/1
  Halin_IMU/1(BHAL_IMU_outputs) -> BHAL_IMU_outputs/1
  VHAL_IMUOffsetVal_raw/1 -> Halin_IMU/1(VHAL_IMUOffsetVal_raw)
  VHAL_IMUOffsetValSta_flg/1 -> Halin_IMU/3(VHAL_IMUOffsetValSta_flg)
  VHAL_IMUSixAxisVal_raw/1 -> Halin_IMU/2(VHAL_IMUSixAxisVal_raw)
  VHAL_IMUSixAxisValSta_flg/1 -> Halin_IMU/4(VHAL_IMUSixAxisValSta_flg)
  VHAL_NvmProtectSta_flg/1 -> Halin_SYS/14(VHAL_NvmProtectSta_flg)
  VHAL_AuxBattVolmV_100mV/1 -> Halin_SYS/15(VHAL_AuxBattVolmV_100mV)
  VHAL_Pedal1Ref5V_raw/1 -> Halin_SYS/16(VHAL_Pedal1Ref5V_raw)
  VHAL_Pedal2Ref5V_raw/1 -> Halin_SYS/17(VHAL_Pedal2Ref5V_raw)
  VHAL_NetworkReqCalled_flg/1 -> Halin_SYS/18(VHAL_NetworkReqCalled_flg)
  VHAL_PmicBootReason_enum/1 -> Halin_SYS/19(VHAL_PmicBootReason_enum)
  VHAL_WisrBootReason_raw32/1 -> Halin_SYS/20(VHAL_WisrBootReason_raw32)
  BHAL_DIDGetData_raw/1 -> Halin_SYS/21(BHAL_DIDGetData_raw)
  VHAL_AcoreRebootCmd_raw/1 -> Halin_SYS/22(VHAL_AcoreRebootCmd_raw)
  VHAL_CAN1BusOff_raw/1 -> Halin_SYS/23(VHAL_CAN1BusOff_raw)
  VHAL_CAN2BusOff_raw/1 -> Halin_SYS/24(VHAL_CAN2BusOff_raw)
  VHAL_CAN3BusOff_raw/1 -> Halin_SYS/25(VHAL_CAN3BusOff_raw)
  VHAL_CAN4BusOff_raw/1 -> Halin_SYS/26(VHAL_CAN4BusOff_raw)
  VHAL_CAN5BusOff_raw/1 -> Halin_SYS/27(VHAL_CAN5BusOff_raw)
  Halin_APM/1(BHAL_APM_outputs) -> BHAL_APM_outputs/1
  u8_TPMSSensorIDRegSta/1 -> Halin_SYS/29(VHAL_TPMSSensorIDRegSta_raw)
  u8_ResetPedalZeroPosReq/1 -> Halin_SYS/30(VHAL_ResetPedalZeroPosReq_raw)
  u8_GetHWIDSta/1 -> Halin_GPIO/17(u8_GetHWIDSta)
  PASDistanceData/1 -> Halin_APM/1(PASDistanceData)
  APSDistanceData/1 -> Halin_APM/2(APSDistanceData)
  APSLevelData/1 -> Halin_APM/3(APSLevelData)
  APSFaultStaData/1 -> Halin_APM/4(APSFaultStaData)
  ChimeIn/1 -> Halin_APM/5(ChimeIn)
  SNSRLayoutIn/1 -> Halin_APM/6(SNSRLayoutIn)
  StaFSyaIn/1 -> Halin_APM/7(StaFSyaIn)
  ModOperationIn/1 -> Halin_APM/8(ModOperationIn)
  u8_GetAPS_Progress_PCT/1 -> Halin_APM/9(u8_GetAPS_Progress_PCT)
  u8_GetAPS_RQ_Display/1 -> Halin_APM/10(u8_GetAPS_RQ_Display)
  u8_GetAPS_SW_Ver/1 -> Halin_APM/11(u8_GetAPS_SW_Ver)
  u8_GetAPS_HW_Ver/1 -> Halin_APM/12(u8_GetAPS_HW_Ver)
  u8_GetAPS_ExitCondition/1 -> Halin_APM/13(u8_GetAPS_ExitCondition)
  f32_GetAPS_Angle_Target/1 -> Halin_APM/14(f32_GetAPS_Angle_Target)
  u8_GetAPS_Sta_System/1 -> Halin_APM/15(u8_GetAPS_Sta_System)
  u8_GetAPS_V_Rq_EPAS_Ctrl/1 -> Halin_APM/16(u8_GetAPS_V_Rq_EPAS_Ctrl)
  u8_GetAPS_Rq_EPAS_Ctrl/1 -> Halin_APM/17(u8_GetAPS_Rq_EPAS_Ctrl)
  u8_GetAPS_Req/1 -> Halin_APM/18(u8_GetAPS_Req)
  f32_GetAPS_DecReq/1 -> Halin_APM/19(f32_GetAPS_DecReq)
  u8_GetAPS_DecReq_A/1 -> Halin_APM/20(u8_GetAPS_DecReq_A)
  f32_GetAPS_SpeedCmd/1 -> Halin_APM/21(f32_GetAPS_SpeedCmd)
  u8_GetAPS_ShftPosnReq/1 -> Halin_APM/22(u8_GetAPS_ShftPosnReq)
  u8_GetAPS_VMC_Req_A/1 -> Halin_APM/23(u8_GetAPS_VMC_Req_A)
  u8_GetCAAS_Sta/1 -> Halin_APM/24(u8_GetCAAS_Sta)
  u8_GetCAAS_VMC_Req_A/1 -> Halin_APM/25(u8_GetCAAS_VMC_Req_A)
  u8_GetAPS_PwrReq_cmd/1 -> Halin_APM/26(u8_GetAPS_PwrReq_cmd)
  u8_GetRAPS_BCM_LockReq_Cmd/1 -> Halin_APM/27(u8_GetRAPS_BCM_LockReq_Cmd)
  u8_GetRAPS_BCM_Lamp_Cmd/1 -> Halin_APM/28(u8_GetRAPS_BCM_Lamp_Cmd)
  u8_GetRAPS_ErrWarn_Sta/1 -> Halin_APM/29(u8_GetRAPS_ErrWarn_Sta)
  u8_GetRAPS_ErrLv1_flg/1 -> Halin_APM/30(u8_GetRAPS_ErrLv1_flg)
  VHAL_CAN6BusOff_raw/1 -> Halin_SYS/28(VHAL_CAN6BusOff_raw)
  u32_BootPath/1 -> Halin_SYS/31(VHAL_PmicBootPath_raw32)
  VHAL_CAN1RxErrorCount_raw/1 -> Halin_SYS/32(VHAL_CAN1RxErrorCount_raw)
  VHAL_CAN1TxErrorCount_raw/1 -> Halin_SYS/33(VHAL_CAN1TxErrorCount_raw)
  VHAL_CAN2RxErrorCount_raw/1 -> Halin_SYS/34(VHAL_CAN2RxErrorCount_raw)
  VHAL_CAN2TxErrorCount_raw/1 -> Halin_SYS/35(VHAL_CAN2TxErrorCount_raw)
  VHAL_CAN3RxErrorCount_cnt/1 -> Halin_SYS/36(VHAL_CAN3RxErrorCount_raw)
  VHAL_CAN3TxErrorCount_raw/1 -> Halin_SYS/37(VHAL_CAN3TxErrorCount_raw)
  VHAL_CAN4RxErrorCount_raw/1 -> Halin_SYS/38(VHAL_CAN4RxErrorCount_raw)
  VHAL_CAN4TxErrorCount_raw/1 -> Halin_SYS/39(VHAL_CAN4TxErrorCount_raw)
  VHAL_CAN5RxErrorCount_raw/1 -> Halin_SYS/40(VHAL_CAN5RxErrorCount_raw)
  VHAL_CAN5TxErrorCount_raw/1 -> Halin_SYS/41(VHAL_CAN5TxErrorCount_raw)
  VHAL_CAN6RxErrorCount_raw/1 -> Halin_SYS/42(VHAL_CAN6RxErrorCount_raw)
  VHAL_CAN6TxErrorCount_raw/1 -> Halin_SYS/43(VHAL_CAN6TxErrorCount_raw)
